simulink library "CRYP_PF_MASTER"  (Simulink 8.5)
settings: Solver=ode45  StartTime=0.0  StopTime=10.0  RelTol=1e-3
libraries: cdsEpicsOut x53, cdsFilt x16, cdsTP x16, VIS_LIB x8, cdsFunctionCall x5, cdsFiltCtrl x4, cdsMuxMatrix x4, cdsEpicsIn x2, lockin x2, QPD x2, cdsRms x2, FOUROSEM_COILOUTF_MASTER x1
(part 3 of 3)

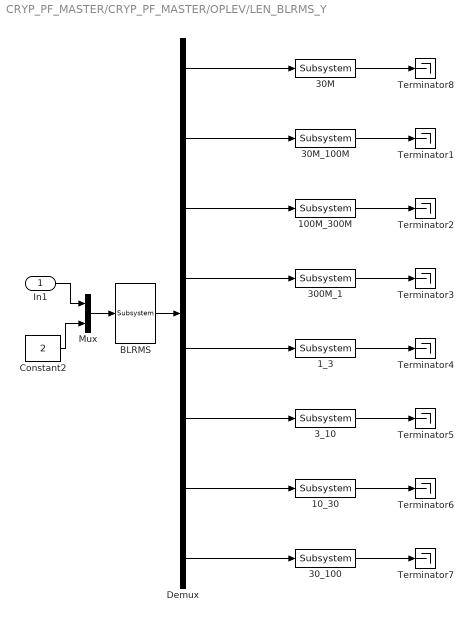
== system CRYP_PF_MASTER/CRYP_PF_MASTER/OPLEV/LEN_BLRMS_Y ==
  In1 : Inport
  100M_300M : cdsEpicsOut/Subsystem  Tag=cdsEpicsOutput  Description=|
      | Purpose:                                          
      | Output a FE signal to an EPICS channel.           
      |                                                   
      | Operation:                                        
      | Takes input value and passes it to EPICS record.  
      |                                                   
      | Usage:                                            
      | Name the part with the desired EPICS rrecord name.
      settings: AttributesFormatString=%<Tag>
  10_30 : cdsEpicsOut/Subsystem  Tag=cdsEpicsOutput  Description=|
      | Purpose:                                          
      | Output a FE signal to an EPICS channel.           
      |                                                   
      | Operation:                                        
      | Takes input value and passes it to EPICS record.  
      |                                                   
      | Usage:                                            
      | Name the part with the desired EPICS rrecord name.
      settings: AttributesFormatString=%<Tag>
  1_3 : cdsEpicsOut/Subsystem  Tag=cdsEpicsOutput  Description=|
      | Purpose:                                          
      | Output a FE signal to an EPICS channel.           
      |                                                   
      | Operation:                                        
      | Takes input value and passes it to EPICS record.  
      |                                                   
      | Usage:                                            
      | Name the part with the desired EPICS rrecord name.
      settings: AttributesFormatString=%<Tag>
  300M_1 : cdsEpicsOut/Subsystem  Tag=cdsEpicsOutput  Description=|
      | Purpose:                                          
      | Output a FE signal to an EPICS channel.           
      |                                                   
      | Operation:                                        
      | Takes input value and passes it to EPICS record.  
      |                                                   
      | Usage:                                            
      | Name the part with the desired EPICS rrecord name.
      settings: AttributesFormatString=%<Tag>
  30M : cdsEpicsOut/Subsystem  Tag=cdsEpicsOutput  Description=|
      | Purpose:                                          
      | Output a FE signal to an EPICS channel.           
      |                                                   
      | Operation:                                        
      | Takes input value and passes it to EPICS record.  
      |                                                   
      | Usage:                                            
      | Name the part with the desired EPICS rrecord name.
      settings: AttributesFormatString=%<Tag>
  30M_100M : cdsEpicsOut/Subsystem  Tag=cdsEpicsOutput  Description=|
      | Purpose:                                          
      | Output a FE signal to an EPICS channel.           
      |                                                   
      | Operation:                                        
      | Takes input value and passes it to EPICS record.  
      |                                                   
      | Usage:                                            
      | Name the part with the desired EPICS rrecord name.
      settings: AttributesFormatString=%<Tag>
  30_100 : cdsEpicsOut/Subsystem  Tag=cdsEpicsOutput  Description=|
      | Purpose:                                          
      | Output a FE signal to an EPICS channel.           
      |                                                   
      | Operation:                                        
      | Takes input value and passes it to EPICS record.  
      |                                                   
      | Usage:                                            
      | Name the part with the desired EPICS rrecord name.
      settings: AttributesFormatString=%<Tag>
  3_10 : cdsEpicsOut/Subsystem  Tag=cdsEpicsOutput  Description=|
      | Purpose:                                          
      | Output a FE signal to an EPICS channel.           
      |                                                   
      | Operation:                                        
      | Takes input value and passes it to EPICS record.  
      |                                                   
      | Usage:                                            
      | Name the part with the desired EPICS rrecord name.
      settings: AttributesFormatString=%<Tag>
  BLRMS : cdsFunctionCall/Subsystem  Tag=cdsFunctionCall  Description=inline BLRMS /opt/rtcds/userapps/release/cds/common/src/BLRMSFILTER.c
      settings: AttributesFormatString=%<Tag>\n%<Description>
  Constant2 : Constant  Value=2
  Demux : Demux  Outputs=8
  Mux : Mux  Inputs=2
  Terminator{1..8} (8 alike) : Terminator
  wires:
  BLRMS/1 -> Demux/1
  Mux/1 -> BLRMS/1
  In1/1 -> Mux/1
  Demux/1 -> 30M/1
  Demux/2 -> 30M_100M/1
  Demux/3 -> 100M_300M/1
  Demux/4 -> 300M_1/1
  Demux/5 -> 1_3/1
  Demux/6 -> 3_10/1
  Demux/7 -> 10_30/1
  Demux/8 -> 30_100/1
  30M/1 -> Terminator8/1
  30M_100M/1 -> Terminator1/1
  100M_300M/1 -> Terminator2/1
  300M_1/1 -> Terminator3/1
  1_3/1 -> Terminator4/1
  3_10/1 -> Terminator5/1
  10_30/1 -> Terminator6/1
  30_100/1 -> Terminator7/1
  Constant2/1 -> Mux/2

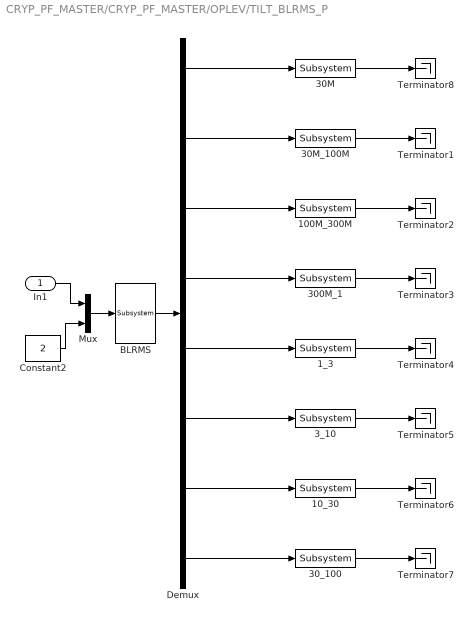
== system CRYP_PF_MASTER/CRYP_PF_MASTER/OPLEV/TILT_BLRMS_P ==
  In1 : Inport
  100M_300M : cdsEpicsOut/Subsystem  Tag=cdsEpicsOutput  Description=|
      | Purpose:                                          
      | Output a FE signal to an EPICS channel.           
      |                                                   
      | Operation:                                        
      | Takes input value and passes it to EPICS record.  
      |                                                   
      | Usage:                                            
      | Name the part with the desired EPICS rrecord name.
      settings: AttributesFormatString=%<Tag>
  10_30 : cdsEpicsOut/Subsystem  Tag=cdsEpicsOutput  Description=|
      | Purpose:                                          
      | Output a FE signal to an EPICS channel.           
      |                                                   
      | Operation:                                        
      | Takes input value and passes it to EPICS record.  
      |                                                   
      | Usage:                                            
      | Name the part with the desired EPICS rrecord name.
      settings: AttributesFormatString=%<Tag>
  1_3 : cdsEpicsOut/Subsystem  Tag=cdsEpicsOutput  Description=|
      | Purpose:                                          
      | Output a FE signal to an EPICS channel.           
      |                                                   
      | Operation:                                        
      | Takes input value and passes it to EPICS record.  
      |                                                   
      | Usage:                                            
      | Name the part with the desired EPICS rrecord name.
      settings: AttributesFormatString=%<Tag>
  300M_1 : cdsEpicsOut/Subsystem  Tag=cdsEpicsOutput  Description=|
      | Purpose:                                          
      | Output a FE signal to an EPICS channel.           
      |                                                   
      | Operation:                                        
      | Takes input value and passes it to EPICS record.  
      |                                                   
      | Usage:                                            
      | Name the part with the desired EPICS rrecord name.
      settings: AttributesFormatString=%<Tag>
  30M : cdsEpicsOut/Subsystem  Tag=cdsEpicsOutput  Description=|
      | Purpose:                                          
      | Output a FE signal to an EPICS channel.           
      |                                                   
      | Operation:                                        
      | Takes input value and passes it to EPICS record.  
      |                                                   
      | Usage:                                            
      | Name the part with the desired EPICS rrecord name.
      settings: AttributesFormatString=%<Tag>
  30M_100M : cdsEpicsOut/Subsystem  Tag=cdsEpicsOutput  Description=|
      | Purpose:                                          
      | Output a FE signal to an EPICS channel.           
      |                                                   
      | Operation:                                        
      | Takes input value and passes it to EPICS record.  
      |                                                   
      | Usage:                                            
      | Name the part with the desired EPICS rrecord name.
      settings: AttributesFormatString=%<Tag>
  30_100 : cdsEpicsOut/Subsystem  Tag=cdsEpicsOutput  Description=|
      | Purpose:                                          
      | Output a FE signal to an EPICS channel.           
      |                                                   
      | Operation:                                        
      | Takes input value and passes it to EPICS record.  
      |                                                   
      | Usage:                                            
      | Name the part with the desired EPICS rrecord name.
      settings: AttributesFormatString=%<Tag>
  3_10 : cdsEpicsOut/Subsystem  Tag=cdsEpicsOutput  Description=|
      | Purpose:                                          
      | Output a FE signal to an EPICS channel.           
      |                                                   
      | Operation:                                        
      | Takes input value and passes it to EPICS record.  
      |                                                   
      | Usage:                                            
      | Name the part with the desired EPICS rrecord name.
      settings: AttributesFormatString=%<Tag>
  BLRMS : cdsFunctionCall/Subsystem  Tag=cdsFunctionCall  Description=inline BLRMS /opt/rtcds/userapps/release/cds/common/src/BLRMSFILTER.c
      settings: AttributesFormatString=%<Tag>\n%<Description>
  Constant2 : Constant  Value=2
  Demux : Demux  Outputs=8
  Mux : Mux  Inputs=2
  Terminator{1..8} (8 alike) : Terminator
  wires:
  BLRMS/1 -> Demux/1
  Mux/1 -> BLRMS/1
  In1/1 -> Mux/1
  Demux/1 -> 30M/1
  Demux/2 -> 30M_100M/1
  Demux/3 -> 100M_300M/1
  Demux/4 -> 300M_1/1
  Demux/5 -> 1_3/1
  Demux/6 -> 3_10/1
  Demux/7 -> 10_30/1
  Demux/8 -> 30_100/1
  30M/1 -> Terminator8/1
  30M_100M/1 -> Terminator1/1
  100M_300M/1 -> Terminator2/1
  300M_1/1 -> Terminator3/1
  1_3/1 -> Terminator4/1
  3_10/1 -> Terminator5/1
  10_30/1 -> Terminator6/1
  30_100/1 -> Terminator7/1
  Constant2/1 -> Mux/2

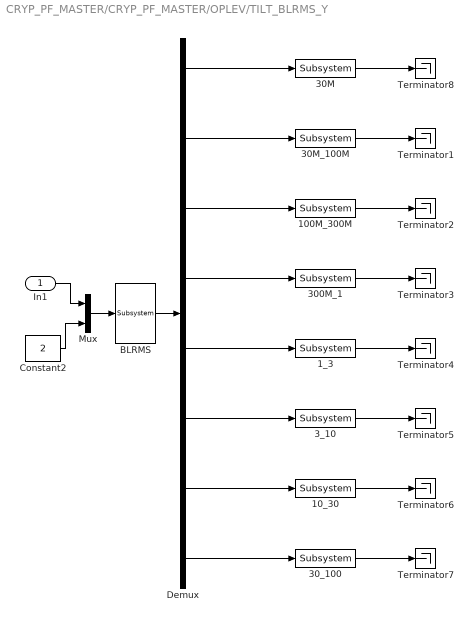
== system CRYP_PF_MASTER/CRYP_PF_MASTER/OPLEV/TILT_BLRMS_Y ==
  In1 : Inport
  100M_300M : cdsEpicsOut/Subsystem  Tag=cdsEpicsOutput  Description=|
      | Purpose:                                          
      | Output a FE signal to an EPICS channel.           
      |                                                   
      | Operation:                                        
      | Takes input value and passes it to EPICS record.  
      |                                                   
      | Usage:                                            
      | Name the part with the desired EPICS rrecord name.
      settings: AttributesFormatString=%<Tag>
  10_30 : cdsEpicsOut/Subsystem  Tag=cdsEpicsOutput  Description=|
      | Purpose:                                          
      | Output a FE signal to an EPICS channel.           
      |                                                   
      | Operation:                                        
      | Takes input value and passes it to EPICS record.  
      |                                                   
      | Usage:                                            
      | Name the part with the desired EPICS rrecord name.
      settings: AttributesFormatString=%<Tag>
  1_3 : cdsEpicsOut/Subsystem  Tag=cdsEpicsOutput  Description=|
      | Purpose:                                          
      | Output a FE signal to an EPICS channel.           
      |                                                   
      | Operation:                                        
      | Takes input value and passes it to EPICS record.  
      |                                                   
      | Usage:                                            
      | Name the part with the desired EPICS rrecord name.
      settings: AttributesFormatString=%<Tag>
  300M_1 : cdsEpicsOut/Subsystem  Tag=cdsEpicsOutput  Description=|
      | Purpose:                                          
      | Output a FE signal to an EPICS channel.           
      |                                                   
      | Operation:                                        
      | Takes input value and passes it to EPICS record.  
      |                                                   
      | Usage:                                            
      | Name the part with the desired EPICS rrecord name.
      settings: AttributesFormatString=%<Tag>
  30M : cdsEpicsOut/Subsystem  Tag=cdsEpicsOutput  Description=|
      | Purpose:                                          
      | Output a FE signal to an EPICS channel.           
      |                                                   
      | Operation:                                        
      | Takes input value and passes it to EPICS record.  
      |                                                   
      | Usage:                                            
      | Name the part with the desired EPICS rrecord name.
      settings: AttributesFormatString=%<Tag>
  30M_100M : cdsEpicsOut/Subsystem  Tag=cdsEpicsOutput  Description=|
      | Purpose:                                          
      | Output a FE signal to an EPICS channel.           
      |                                                   
      | Operation:                                        
      | Takes input value and passes it to EPICS record.  
      |                                                   
      | Usage:                                            
      | Name the part with the desired EPICS rrecord name.
      settings: AttributesFormatString=%<Tag>
  30_100 : cdsEpicsOut/Subsystem  Tag=cdsEpicsOutput  Description=|
      | Purpose:                                          
      | Output a FE signal to an EPICS channel.           
      |                                                   
      | Operation:                                        
      | Takes input value and passes it to EPICS record.  
      |                                                   
      | Usage:                                            
      | Name the part with the desired EPICS rrecord name.
      settings: AttributesFormatString=%<Tag>
  3_10 : cdsEpicsOut/Subsystem  Tag=cdsEpicsOutput  Description=|
      | Purpose:                                          
      | Output a FE signal to an EPICS channel.           
      |                                                   
      | Operation:                                        
      | Takes input value and passes it to EPICS record.  
      |                                                   
      | Usage:                                            
      | Name the part with the desired EPICS rrecord name.
      settings: AttributesFormatString=%<Tag>
  BLRMS : cdsFunctionCall/Subsystem  Tag=cdsFunctionCall  Description=inline BLRMS /opt/rtcds/userapps/release/cds/common/src/BLRMSFILTER.c
      settings: AttributesFormatString=%<Tag>\n%<Description>
  Constant2 : Constant  Value=2
  Demux : Demux  Outputs=8
  Mux : Mux  Inputs=2
  Terminator{1..8} (8 alike) : Terminator
  wires:
  BLRMS/1 -> Demux/1
  Mux/1 -> BLRMS/1
  In1/1 -> Mux/1
  Demux/1 -> 30M/1
  Demux/2 -> 30M_100M/1
  Demux/3 -> 100M_300M/1
  Demux/4 -> 300M_1/1
  Demux/5 -> 1_3/1
  Demux/6 -> 3_10/1
  Demux/7 -> 10_30/1
  Demux/8 -> 30_100/1
  30M/1 -> Terminator8/1
  30M_100M/1 -> Terminator1/1
  100M_300M/1 -> Terminator2/1
  300M_1/1 -> Terminator3/1
  1_3/1 -> Terminator4/1
  3_10/1 -> Terminator5/1
  10_30/1 -> Terminator6/1
  30_100/1 -> Terminator7/1
  Constant2/1 -> Mux/2

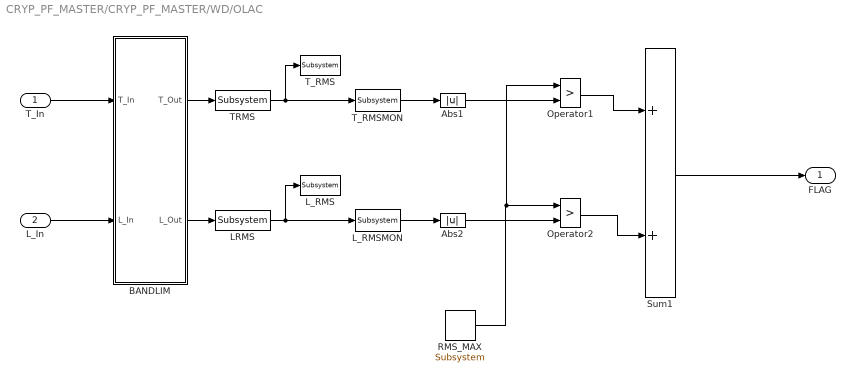
== system CRYP_PF_MASTER/CRYP_PF_MASTER/WD/OLAC ==
  T_In : Inport
  L_In : Inport  Port=2
  Abs1 : Abs
  Abs2 : Abs
  BANDLIM : Subsystem
  LRMS : cdsRms/Subsystem  Tag=cdsRms  Description=|
      | Purpose:
      | Calculate an RMS based on the input signal.
      settings: AttributesFormatString=%<Tag>
  L_RMS : cdsTP/Subsystem  Tag=Test Point
      settings: AttributesFormatString=%<Tag>
  L_RMSMON : cdsEpicsOut/Subsystem  Tag=cdsEpicsOutput  Description=|
      | Purpose:                                          
      | Output a FE signal to an EPICS channel.           
      |                                                   
      | Operation:                                        
      | Takes input value and passes it to EPICS record.  
      |                                                   
      | Usage:                                            
      | Name the part with the desired EPICS rrecord name.
      settings: AttributesFormatString=%<Tag>
  Operator1 : RelationalOperator  Operator=>  OutDataTypeStr=boolean
  Operator2 : RelationalOperator  Operator=>  OutDataTypeStr=boolean
  RMS_MAX : cdsEpicsIn/Subsystem  Tag=cdsEpicsIn  Description=|
      | Purpose:                                                                              
      | Create an EPICS input channel connection to the FE realtime controls.                 
      |                                                                                       
      | Operation:                                                                            
      | Outputs value from an EPICS ai record. Value is floating point with a precision of 3..
      |                                                                                       
      | Usage:                                                                                
      | Name the part with the desired EPICS channel name.
      settings: AttributesFormatString=%<Tag>
  Sum1 : Sum
  TRMS : cdsRms/Subsystem  Tag=cdsRms  Description=|
      | Purpose:
      | Calculate an RMS based on the input signal.
      settings: AttributesFormatString=%<Tag>
  T_RMS : cdsTP/Subsystem  Tag=Test Point
      settings: AttributesFormatString=%<Tag>
  T_RMSMON : cdsEpicsOut/Subsystem  Tag=cdsEpicsOutput  Description=|
      | Purpose:                                          
      | Output a FE signal to an EPICS channel.           
      |                                                   
      | Operation:                                        
      | Takes input value and passes it to EPICS record.  
      |                                                   
      | Usage:                                            
      | Name the part with the desired EPICS rrecord name.
      settings: AttributesFormatString=%<Tag>
  FLAG : Outport
  wires:
  Sum1/1 -> FLAG/1
  TRMS/1 -> T_RMSMON/1, T_RMS/1
  LRMS/1 -> L_RMSMON/1, L_RMS/1
  RMS_MAX/1 -> Operator1/1, Operator2/1
  Abs2/1 -> Operator2/2
  Operator2/1 -> Sum1/2
  Operator1/1 -> Sum1/1
  T_RMSMON/1 -> Abs1/1
  L_RMSMON/1 -> Abs2/1
  T_In/1 -> BANDLIM/1(T_In)
  L_In/1 -> BANDLIM/2(L_In)
  BANDLIM/1(T_Out) -> TRMS/1
  BANDLIM/2(L_Out) -> LRMS/1
  Abs1/1 -> Operator1/2

== system CRYP_PF_MASTER/CRYP_PF_MASTER/WD/OLAC/BANDLIM ==
  T_In : Inport
  L_In : Inport  Port=2
  L : cdsFilt/Subsystem  Tag=cdsFilt  Description=|
      | Purpose:                                                                                                                                                                                                                                  
      | Standard CDS IIR filter module.                                                                                                                                                                                                           
      |                                                                                                                                                                                                                                           
      | Operation:                                                                                                                                                                                                                                
      | Consists of 10 second order section IIR filters, plus a ramped gain stage. In FE code, also provides pre-defined test points and excitation channel inputs. The filter coefficients are defined in the LIGO system using the 'foton' tool.
      |                                                                                                                                                                                                                                           
      | Usage:                                                                                                                                                                                                                                    
      | Name the part with the desired filter module name.
      settings: AttributesFormatString=%<Tag>
  T : cdsFilt/Subsystem  Tag=cdsFilt  Description=|
      | Purpose:                                                                                                                                                                                                                                  
      | Standard CDS IIR filter module.                                                                                                                                                                                                           
      |                                                                                                                                                                                                                                           
      | Operation:                                                                                                                                                                                                                                
      | Consists of 10 second order section IIR filters, plus a ramped gain stage. In FE code, also provides pre-defined test points and excitation channel inputs. The filter coefficients are defined in the LIGO system using the 'foton' tool.
      |                                                                                                                                                                                                                                           
      | Usage:                                                                                                                                                                                                                                    
      | Name the part with the desired filter module name.
      settings: AttributesFormatString=%<Tag>
  T_Out : Outport
  L_Out : Outport  Port=2
  wires:
  T/1 -> T_Out/1
  L/1 -> L_Out/1
  T_In/1 -> T/1
  L_In/1 -> L/1
